simulink model "rw_model"  (R2019b)
settings: Solver=VariableStepAuto  StartTime=0.0  StopTime=600  RelTol=1e-3
undefined symbols (not defined in the file or in its folder): c, I, J, Kd, Ki, Kp, N, R
settings Model: Creator=asmialek  LastModifiedBy=asmialek
settings DataIOCC: SaveOutput=off  SignalLogging=off  DSMLogging=off  ReturnWorkspaceOutputs=off

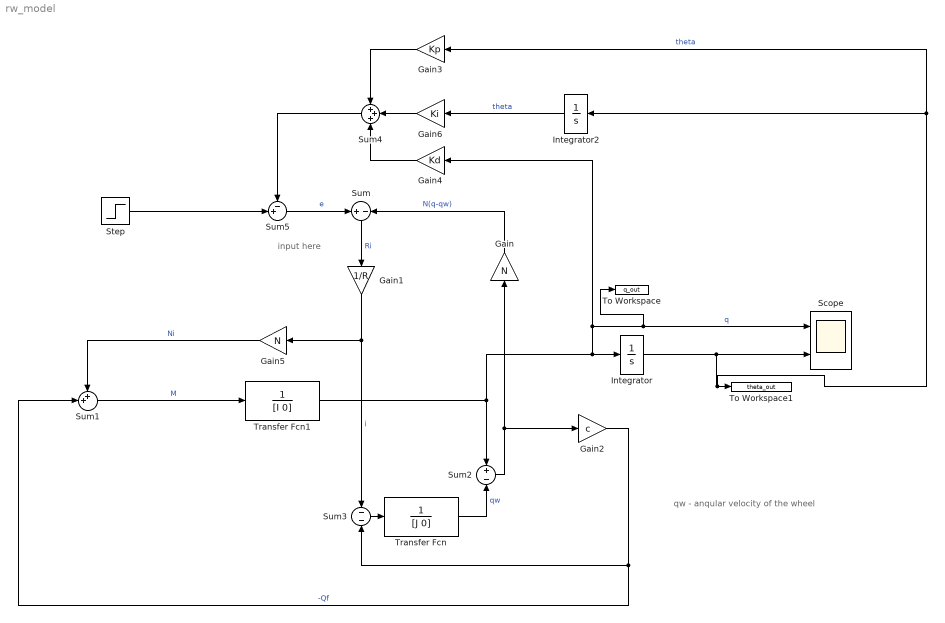
== system rw_model ==
  note: qw - anqular velocity of the wheel
  note: input here
  Gain : Gain  Gain=N
  Gain1 : Gain  Gain=1/R
  Gain2 : Gain  Gain=c
  Gain3 : Gain  Gain=Kp
  Gain4 : Gain  Gain=Kd
  Gain5 : Gain  Gain=N
  Gain6 : Gain  Gain=Ki
  Integrator : Integrator
  Integrator2 : Integrator
  Scope : Scope  NumInputPorts=2
  Step : Step  Time=20  After=5  SampleTime=0
  Sum : Sum  Inputs=+|-
  Sum1 : Sum  Inputs=++|
  Sum2 : Sum  Inputs=+|-
  Sum3 : Sum  Inputs=-|-
  Sum4 : Sum  Inputs=+++
  Sum5 : Sum  Inputs=-+|
  To Workspace : ToWorkspace  VariableName=q_out  SampleTime=-1
  To Workspace1 : ToWorkspace  VariableName=theta_out  SampleTime=-1
  Transfer Fcn : TransferFcn  Denominator=[J 0]
  Transfer Fcn1 : TransferFcn  Denominator=[I 0]
  wires:
  Transfer Fcn1/1 -> Integrator/1, Gain4/1, To Workspace/1, Scope/1, Sum2/1  "q"
  Gain/1 -> Sum/2  "N(q-qw)"
  Sum/1 -> Gain1/1  "Ri"
  Gain1/1 -> Sum3/1, Gain5/1  "i"
  Transfer Fcn/1 -> Sum2/2  "qw"
  Sum2/1 -> Gain/1, Gain2/1
  Gain2/1 -> Sum3/2, Sum1/2  "-Qf"
  Gain3/1 -> Sum4/1
  Sum5/1 -> Sum/1  "e"
  Step/1 -> Sum5/2
  Sum4/1 -> Sum5/1
  Gain5/1 -> Sum1/1  "Ni"
  Sum1/1 -> Transfer Fcn1/1  "M"
  Gain4/1 -> Sum4/3
  Integrator2/1 -> Gain6/1  "theta"
  Gain6/1 -> Sum4/2
  Integrator/1 -> Gain3/1, Integrator2/1, To Workspace1/1, Scope/2  "theta"
  Sum3/1 -> Transfer Fcn/1
